simulink model "a6"  (R2021a)
settings: Solver=VariableStepAuto  StartTime=0.0  StopTime=2  RelTol=1e-3
undefined symbols (not defined in the file or in its folder): Down, Up
libraries: spsSeriesRLCBranchLib x4, eePwmGenerator x2, spsDiodeLib x2, powerlib_extras x1, spsPVArrayLib x1, spsIGBTDiodeLib x1, spsVoltageMeasurementLib x1, spspowerguiLib x1
settings Model: Creator=Dell  LastModifiedBy=Dell

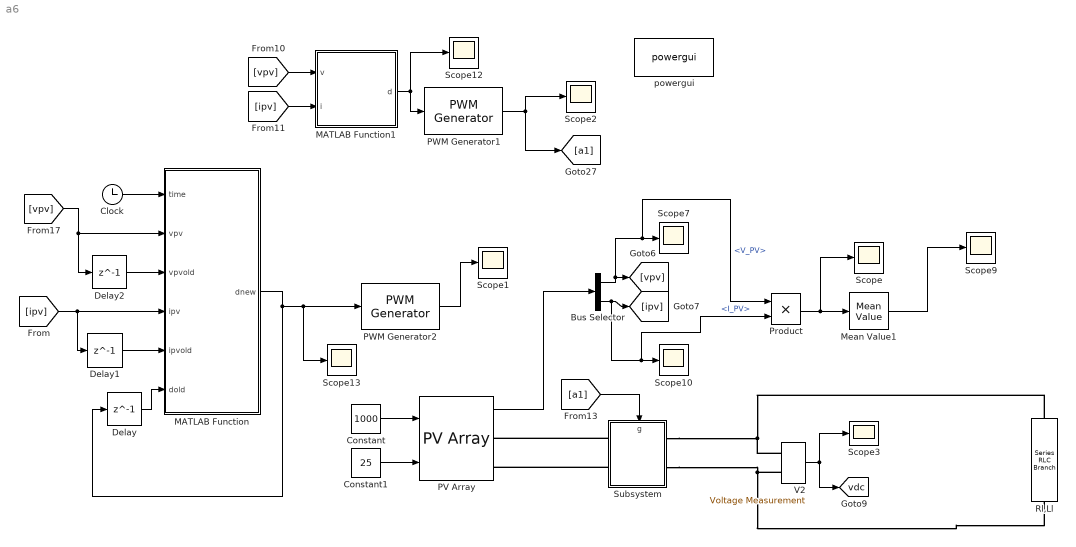
== system a6 ==
  Bus Selector : BusSelector  OutputSignals=V_PV,I_PV
  Clock : Clock
  Constant : Constant  Value=1000
  Constant1 : Constant  Value=25
  Delay : Delay  DelayLength=1
  Delay1 : Delay  DelayLength=1
  Delay2 : Delay  DelayLength=1
  MATLAB Function : MATLAB Function  TreatAsAtomicUnit=on
  MATLAB Function1 : MATLAB Function  TreatAsAtomicUnit=on
  Mean Value1 : powerlib_extras/Measurements/Mean Value  Period=1/100
      settings: SourceProductBaseCode=PS
  PV Array : spsPVArrayLib/PV Array  Npar=1  Nser=6  PlotType=array @ 1000 W/m2 & specified temperatures  S_vec="[ 1000  500  100 ]"  Temp_C_vec=[ 25 ]  ModuleName=User-defined  PlotWhenSelected=off  Pm=335.28  Ncell=60  Voc=46.8  Isc=9.3  Vm=38.1  Im=8.8  beta_Voc_pc=-0.36099  alpha_Isc_pc=0.102  beta_Voc=-0.16894  alpha_Isc=0.009486  IL=9.3302  I0=3.4457e-10  nI=1.2642  Rsh=710.4206  Rs=0.33548  RobustModel=off  RobustCellTemperature=313.3991  BAL=on  Tc=1e-6  Tfilter=5e-5
  PWM Generator1 : eePwmGenerator/PWM Generator  CarrCount=Up-Down  Tper=1/15000  Ts=5e-6
  PWM Generator2 : eePwmGenerator/PWM Generator  CarrCount=Up  Tper=1/15000  Ts=5e-6
  Product : Product
  Rl,Ll : spsSeriesRLCBranchLib/Series RLC Branch  LConnTagsString=__new0  RConnTagsString=__new0  BranchType=R  Resistance=1000  Inductance=25e-3  SetiL0=off  InitialCurrent=0  Capacitance=1.0  Setx0=off  InitialVoltage=0  Measurements=None
  Scope{,1..3,7,9..10,12..13} (9 alike) : Scope
  Subsystem : Subsystem
      settings: PortSchema="{\"entries\":[{\"content\":{\"sides\":[{\"content\":{\"connectorIds\":[\"LConn1\",\"LConn2\"]},\"type\":\"ConnectorPlacement.EquallySpacedRectSide\",\"uuid\":\"8d150eef-90b5-4fdb-be84-a9f6f4ebd895\"},{\"content\":{\"connectorIds\":[\"RConn1\",\"RConn2\"],\"side\":\"RIGHT\"},\"type\":\"ConnectorPlacement.EquallySpacedRectSide\",\"uuid\":\"8602e169-ea88-4412-9b25-fadbb117dfcf\"},{\"content\":{\"connectorIds\":[\"In1\"],\"side\":\"TOP\"},\"type\":\"ConnectorPlacement.EquallySpacedRectSide\",\"uuid\":\"8809c1af-ab1c-4eed-b81f-f8f2792471ea\"}]},\"type\":\"ConnectorPlacement.EquallySpacedConnector\",\"uuid\":\"c77f0f7f-21b7-47e6-a535-29cdb02ea9e2\"}],\"packageUris\":[\"http://schema.mathworks.com/mf0/Connector/R2020b\"],\"version\":\"1.0\"}"
  V2 : spsVoltageMeasurementLib/Voltage Measurement  PhasorSimulation=off  OutputType=Complex  PSBequivalent=0
  powergui : spspowerguiLib/powergui  Priority=1  SimulationMode=Discrete  SampleTime=5e-6  frequency=60  Iterations=50  frequencyindice=0  Pbase=100e6  ErrMax=1e-4  UnitsV=kV  UnitsW=MW  buscounter=0  FunctionMessages=off  echomessages=off  EnableUseOfTLC=off  CurrentSourceSwitches=off  DisableSnubberDevices=off  DisableRonSwitches=off  DisableVfSwitches=off  DisplayEquations=off  AutomaticDiscreteSolvers=off  SolverType=Tustin/Backward Euler (TBE)  Interpol=off  ExternalGateDelay=off  methode=off  Ts=100  x0status=blocks  SPID=on  SwTol=0  HookPort=off  NonlinearTolerance=1e-4  nMaxIteration=100  ContinueOnMaxIteration=off  RestoreLinks=warning  ResistiveCurrentMeasurement=off  Frange=[0:2:500]  Ylog=off  Xlog=on  ShowGrid=off  save=off  variable=ZData  structure=0  ZoomFFT=off  StartTime=0.0  cycles=1  DisplayStyle=1  fundamental=60  FreqAxis=off  MaxFrequency=1000  frequencyindicesteady=1  RmsSteady=1  display=off
  tag scope: vdc=global
  wires:
  V2/1 -> [vdc], Scope3/1
  Constant1/1 -> PV Array/2
  Constant/1 -> PV Array/1
  Bus Selector/2 -> Product/2, Scope10/1, [ipv]  "<I_PV>"
  Bus Selector/1 -> Product/1, Scope7/1, [vpv]  "<V_PV>"
  PV Array/1 -> Bus Selector/1
  Mean Value1/1 -> Scope9/1
  Product/1 -> Scope/1, Mean Value1/1
  [a1] -> Subsystem/1(g)
  MATLAB Function/1(dnew) -> PWM Generator2/1, Scope13/1, Delay/1
  [vpv] -> MATLAB Function/2(vpv), Delay2/1
  Delay2/1 -> MATLAB Function/3(vpvold)
  [ipv] -> Delay1/1, MATLAB Function/4(ipv)
  Delay/1 -> MATLAB Function/6(dold)
  Delay1/1 -> MATLAB Function/5(ipvold)
  MATLAB Function1/1(d) -> Scope12/1, PWM Generator1/1
  [vpv] -> MATLAB Function1/1(v)
  [ipv] -> MATLAB Function1/2(i)
  PWM Generator2/1 -> Scope1/1
  Clock/1 -> MATLAB Function/1(time)
  PWM Generator1/1 -> Scope2/1, [a1]
  connections:
  Rl,Ll/LConn1 -- V2/LConn1 -- Subsystem/RConn1
  V2/LConn2 -- Subsystem/RConn2 -- Rl,Ll/RConn1
  Subsystem/LConn2 -- PV Array/RConn2
  Subsystem/LConn1 -- PV Array/RConn1

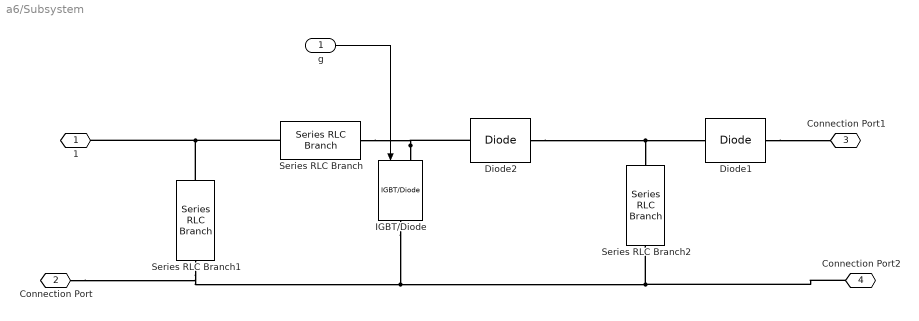
== system a6/Subsystem ==
  g : Inport
  Diode1 : spsDiodeLib/Diode  Ron=0.001  Lon=0  Vf=0.8  IC=0  UseSnubber=0  Rs=0  Cs=0  Measurements=off
  Diode2 : spsDiodeLib/Diode  Ron=0.001  Lon=0  Vf=0.8  IC=0  UseSnubber=0  Rs=0  Cs=0  Measurements=off
  IGBT/Diode : spsIGBTDiodeLib/IGBT//Diode  Ron=1e-3  Rs=1e5  Cs=inf  Measurements=off
  Series RLC Branch : spsSeriesRLCBranchLib/Series RLC Branch  LConnTagsString=__new0  RConnTagsString=__new0  BranchType=L  Resistance=1  Inductance=5e-3  SetiL0=off  InitialCurrent=0  Capacitance=1e-6  Setx0=off  InitialVoltage=0  Measurements=None
  Series RLC Branch1 : spsSeriesRLCBranchLib/Series RLC Branch  LConnTagsString=__new0  RConnTagsString=__new0  BranchType=C  Resistance=1  Inductance=1e-3  SetiL0=off  InitialCurrent=0  Capacitance=1100e-6  Setx0=off  InitialVoltage=0  Measurements=None
  Series RLC Branch2 : spsSeriesRLCBranchLib/Series RLC Branch  LConnTagsString=__new0  RConnTagsString=__new0  BranchType=C  Resistance=1  Inductance=1e-3  SetiL0=off  InitialCurrent=0  Capacitance=1100e-6  Setx0=off  InitialVoltage=0  Measurements=None
  1 : PMIOPort  Side=Left
  Connection Port : PMIOPort  Port=2  Side=Left
  Connection Port1 : PMIOPort  Port=3  Side=Right
  Connection Port2 : PMIOPort  Port=4  Side=Right
  wires:
  g/1 -> IGBT/Diode/1
  connections:
  IGBT/Diode/LConn1 -- Series RLC Branch/RConn1 -- Diode2/LConn1
  IGBT/Diode/RConn1 -- Connection Port/RConn1 -- Series RLC Branch1/RConn1 -- Connection Port2/RConn1 -- Series RLC Branch2/RConn1
  Diode2/RConn1 -- Diode1/LConn1 -- Series RLC Branch2/LConn1
  Diode1/RConn1 -- Connection Port1/RConn1
  Series RLC Branch/LConn1 -- 1/RConn1 -- Series RLC Branch1/LConn1

== matlab function a6/MATLAB Function1 ==
  data: v input; d output; i input
function d = fcn(v,i)

persistent vprev;
persistent dprev;
persistent pprev;

if isempty(vprev)
    vprev=0;
end
if isempty(dprev)
    dprev=0;
end
if isempty(pprev)
    pprev=0;
end

d = dprev;
p = v*i;
deltav = v - vprev;
deltap = p -pprev;
k = 0.1;

if deltap>0
    if deltav>0
        d = dprev - k;
    elseif deltav <0
        d = dprev + k;
    end
elseif deltap<0
    if deltav>0
        d = dprev + k;
    elseif deltav<0
        d = dprev - k;
    end
end

if d>0.9
    d=0.9;
elseif d<0
    d=0;
end
vprev = v;
pprev = p;
dprev = d;

== matlab function a6/MATLAB Function ==
  data: time input; vpv input; dnew output; vpvold input; ipv input; ipvold input; dold input
function dnew = fcn(time,vpv,vpvold,ipv,ipvold,dold)
k=0.0001;
dstart = 0.05 ;
ppv = vpv * ipv;
ppvold = vpvold * ipvold;
if time<0.6
    dnew = dstart;
else
    if(ppv == ppvold)
    dnew = dold;
    else
        if(ppv > ppvold)
            if(vpv>vpvold)
                dnew=dold-k;
            else
                dnew = dold+k;
            end
        else
           if(vpv>vpvold)
              dnew = dold+k;
           else
              dnew=dold-k;
           end
        end
    end
end    
if dnew>0.95
    dnew = 0.94;
else
    if dnew < 0.15
        dnew = 0.16;
    end
end
